simulink model "observer_state"  (R2015a)
settings: Solver=ode45  StartTime=0.0  StopTime=10  FixedStep=1e-6  RelTol=1e-3
values from neighbouring files (symbols this model uses):
  a = [0 1;0 0]    [ejemplo_jury.m]    (also in observer_minimum.m = [0 1;0 -1]; realim_state_pd.m = [0 1;0 -1])
  b = [0;1]    [ejemplo_jury.m]    (also in observer_minimum.m = [0; 10]; realim_state_pd.m = [0; 10])
  c = [1 0]    [ejemplo_jury.m]    (also in observer_minimum.m; realim_state_pd.m)
  d = 0    [ejemplo_jury.m]    (also in observer_minimum.m; realim_state_pd.m)
  k1 = 2.39    [ejemplo_jury.m]    (also in observer_minimum.m = [8.8 2.3]; realim_state_pd.m = [8.8 2.3])
  k2 = 16    [observer_minimum.m]    (also in realim_state_pd.m)
  Ko_corr_2 = [149; 4851]    [realim_state_pd.m]
settings Model: Creator=Jose Roldan  LastModifiedBy=Jose Roldan

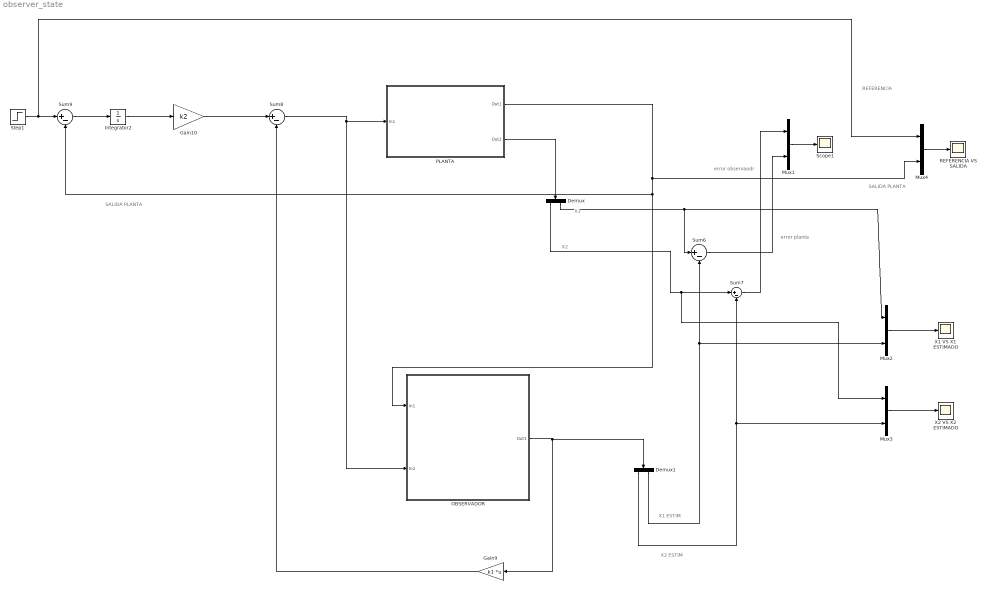
== system observer_state ==
  note: X2 ESTIM
  note: X1 ESTIM
  note: SALIDA PLANTA
  note: REFERENCIA
  note: SALIDA PLANTA
  note: X2
  note: X1
  note: error observaodr
  note: error planta
  Demux : Demux  Outputs=2
  Demux1 : Demux  Outputs=2
  Gain10 : Gain  Gain=k2
  Gain9 : Gain  Gain=k1  Multiplication=Matrix(K*u)
  Integrator2 : Integrator
  Mux{1..4} (4 alike) : Mux  Inputs=2
  OBSERVADOR : Subsystem
  PLANTA : Subsystem
  REFERENCIA VS SALIDA : Scope
      settings: SaveName=ScopeData3
  Scope1 : Scope
  Step1 : Step  Time=0  SampleTime=0
  Sum{6..9} (4 alike) : Sum  Inputs=|+-
  X1 VS X1 ESTIMADO : Scope
  X2 VS X2 ESTIMADO : Scope
      settings: SaveName=ScopeData2
  wires:
  Mux1/1 -> Scope1/1
  Demux/2 -> Sum6/1, Mux2/1
  Demux/1 -> Mux3/1, Sum7/1
  Sum6/1 -> Mux1/2
  Sum8/1 -> PLANTA/1(In1), OBSERVADOR/2(In2)
  Sum7/1 -> Mux1/1
  Mux2/1 -> X1 VS X1 ESTIMADO/1
  Mux3/1 -> X2 VS X2 ESTIMADO/1
  Gain10/1 -> Sum8/1
  Gain9/1 -> Sum8/2
  Mux4/1 -> REFERENCIA VS SALIDA/1
  Step1/1 -> Mux4/1, Sum9/1
  Sum9/1 -> Integrator2/1
  Integrator2/1 -> Gain10/1
  OBSERVADOR/1(Out3) -> Demux1/1, Gain9/1
  Demux1/2 -> Mux2/2, Sum6/2
  Demux1/1 -> Mux3/2, Sum7/2
  PLANTA/1(Out1) -> OBSERVADOR/1(In1), Sum9/2, Mux4/2
  PLANTA/2(Out2) -> Demux/1

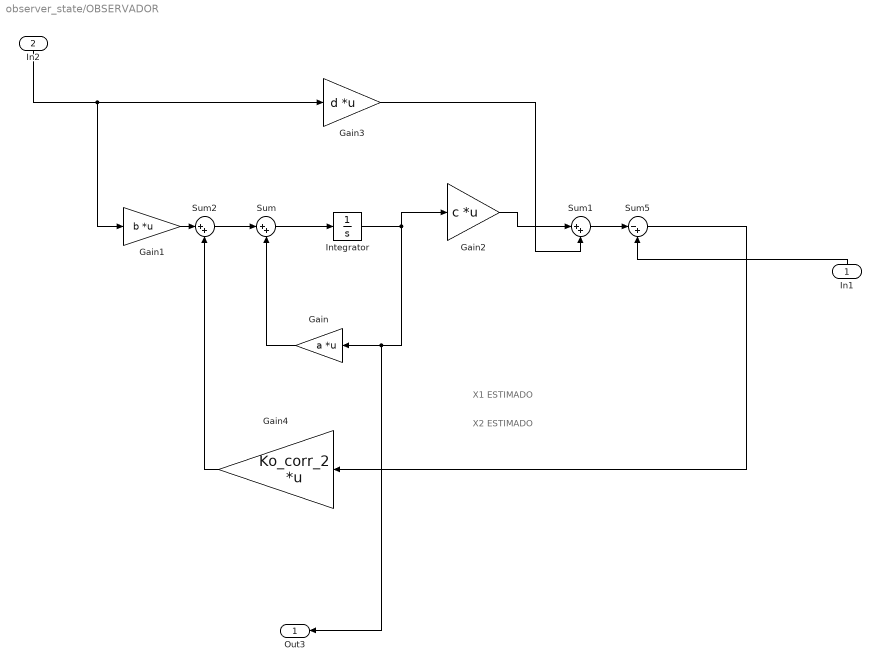
== system observer_state/OBSERVADOR ==
  note: X2 ESTIMADO
  note: X1 ESTIMADO
  In1 : Inport
  In2 : Inport  Port=2
  Gain : Gain  Gain=a  Multiplication=Matrix(K*u)
  Gain1 : Gain  Gain=b  Multiplication=Matrix(K*u)
  Gain2 : Gain  Gain=c  Multiplication=Matrix(K*u)
  Gain3 : Gain  Gain=d  Multiplication=Matrix(K*u)
  Gain4 : Gain  Gain=Ko_corr_2  Multiplication=Matrix(K*u)
  Integrator : Integrator
  Sum : Sum  Inputs=|++
  Sum1 : Sum  Inputs=|++
  Sum2 : Sum  Inputs=|++
  Sum5 : Sum  Inputs=|-+
  Out3 : Outport
  wires:
  In2/1 -> Gain3/1, Gain1/1
  In1/1 -> Sum5/2
  Sum/1 -> Integrator/1
  Integrator/1 -> Gain2/1, Out3/1, Gain/1
  Gain/1 -> Sum/2
  Gain2/1 -> Sum1/1
  Gain1/1 -> Sum2/1
  Gain3/1 -> Sum1/2
  Gain4/1 -> Sum2/2
  Sum2/1 -> Sum/1
  Sum5/1 -> Gain4/1
  Sum1/1 -> Sum5/1

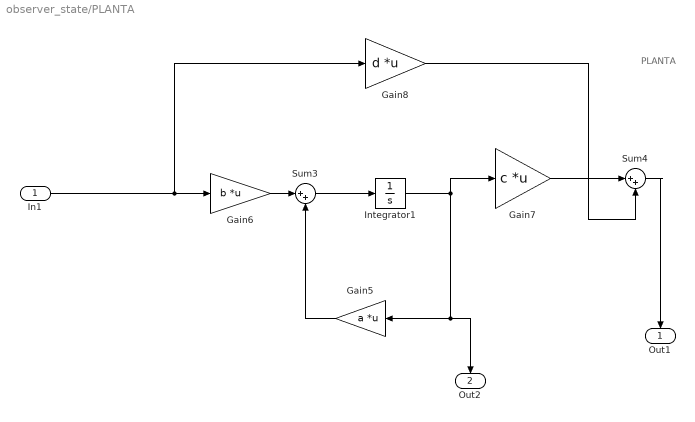
== system observer_state/PLANTA ==
  note: PLANTA
  In1 : Inport
  Gain5 : Gain  Gain=a  Multiplication=Matrix(K*u)
  Gain6 : Gain  Gain=b  Multiplication=Matrix(K*u)
  Gain7 : Gain  Gain=c  Multiplication=Matrix(K*u)
  Gain8 : Gain  Gain=d  Multiplication=Matrix(K*u)
  Integrator1 : Integrator
  Sum3 : Sum  Inputs=|++
  Sum4 : Sum  Inputs=|++
  Out1 : Outport
  Out2 : Outport  Port=2
  wires:
  In1/1 -> Gain8/1, Gain6/1
  Sum4/1 -> Out1/1
  Gain7/1 -> Sum4/1
  Sum3/1 -> Integrator1/1
  Gain5/1 -> Sum3/2
  Gain8/1 -> Sum4/2
  Gain6/1 -> Sum3/1
  Integrator1/1 -> Gain7/1, Out2/1, Gain5/1
